simulink model "sensor_less"  (R2023a)
settings: Solver=VariableStepAuto  StartTime=0.0  StopTime=1  RelTol=1e-3
libraries: spsMosfetLib x6, slpidlib x1, spsPermanentMagnetSynchronousMachineLib x1, spsDCVoltageSourceLib x1, dspswit3 x1, spspowerguiLib x1
settings Model: Creator=heman  LastModifiedBy=ANKIT
settings SolverCC: ZeroCrossAlgorithm=Adaptive
settings DebuggingCC: IgnoredZcDiagnostic=none

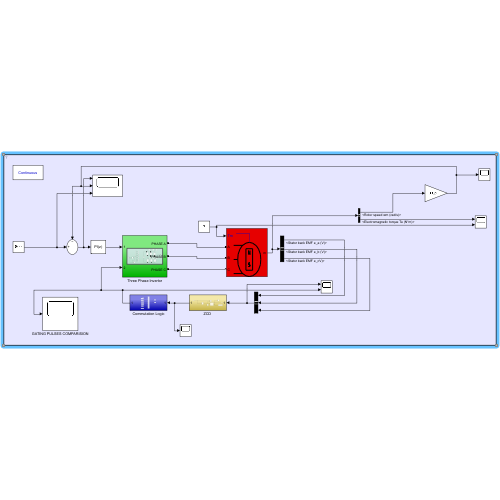
[thumbnail: Simulink's stored preview of the top-level diagram]
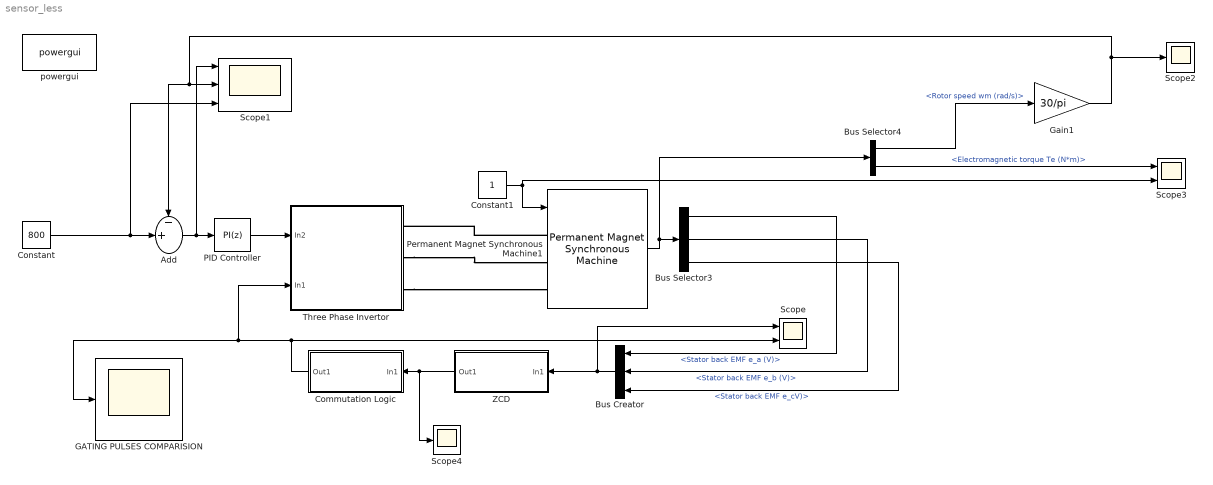
== system sensor_less ==
  Add : Sum  Inputs=-+|
  Bus Creator : BusCreator  Inputs=3
  Bus Selector3 : BusSelector  OutputSignals=Stator back EMF e_a (V),Stator back EMF e_b (V),Stator back EMF e_cV)
  Bus Selector4 : BusSelector  OutputSignals=Rotor speed wm (rad/s),Electromagnetic torque Te (N*m)
  Commutation Logic : Subsystem
  Constant : Constant  Value=800
  Constant1 : Constant
  GATING PULSES COMPARISION : Scope
  Gain1 : Gain  Gain=30/pi
  PID Controller : slpidlib/PID Controller  Controller=PI  Form=Parallel  TimeDomain=Discrete-time  UseExternalTs=off  SampleTime=-1  IntegratorMethod=Forward Euler  FilterMethod=Forward Euler  ControllerParametersSource=internal  P=0.01035  I=12.77  UseKiTs=on  D=500  N=100  UseFilter=on  TunerSelectOption=Frequency Response Based  InitialConditionSource=internal  InitialConditionForIntegrator=0  InitialConditionForFilter=0  DifferentiatorICPrevScaledInput=0  ExternalReset=none  TrackingMode=off  Kt=1  LimitOutput=off  SatLimitsSource=internal  UpperSaturationLimit=inf  LowerSaturationLimit=-inf  LinearizeAsGain=on  AntiWindupMode=none  Kb=1  LimitIntegrator=off  UpperIntegratorSaturationLimit=inf  LowerIntegratorSaturationLimit=-inf  POutMin=[]  POutMax=[]  IOutMin=[]  IOutMax=[]  DOutMin=[]  DOutMax=[]  NOutMin=[]  NOutMax=[]  SumOutMin=[]  SumOutMax=[]  SaturationOutMin=[]  SaturationOutMax=[]  PParamMin=[]  PParamMax=[]  IParamMin=[]  IParamMax=[]  DParamMin=[]  DParamMax=[]  NParamMin=[]  NParamMax=[]  KbParamMin=[]  KbParamMax=[]  KtParamMin=[]  KtParamMax=[]  KbOutMin=[]  KbOutMax=[]  KtOutMin=[]  KtOutMax=[]  IntegratorOutMin=[]  IntegratorOutMax=[]  FilterOutMin=[]  FilterOutMax=[]  SumI1OutMin=[]  SumI1OutMax=[]  SumI2OutMin=[]  SumI2OutMax=[]  SumI3OutMin=[]  SumI3OutMax=[]  SumI4OutMin=[]  SumI4OutMax=[]  SumDOutMin=[]  SumDOutMax=[]  DifferentiatorOutMin=[]  DifferentiatorOutMax=[]  FilterDiffOutCoefMin=[]  FilterDiffOutCoefMax=[]  ReciprocalOutMin=[]  ReciprocalOutMax=[]  SumDenOutMin=[]  SumDenOutMax=[]  SumNumOutMin=[]  SumNumOutMax=[]  DivideOutMin=[]  DivideOutMax=[]  UdiffTsProdOutMin=[]  UdiffTsProdOutMax=[]  NTsProdOutMin=[]  NTsProdOutMax=[]  UintegralTsProdOutMin=[]  UintegralTsProdOutMax=[]  UngainTsProdOutMin=[]  UngainTsProdOutMax=[]  ClampingZeroOutDataTypeStr=Inherit: Inherit via back propagation  ClampingZeroOutMin=[]  ClampingZeroOutMax=[]  FilterDenConstantOutDataTypeStr=Inherit: Inherit via back propagation  FilterDenConstantOutMin=[]  FilterDenConstantOutMax=[]  PCopyOutDataTypeStr=Inherit: Inherit via back propagation  PCopyOutMin=[]  PCopyOutMax=[]  NCopyOutDataTypeStr=Inherit: Inherit via back propagation  NCopyOutMin=[]  NCopyOutMax=[]  IntegratorContinuousStateAttributes=''  IntegratorStateMustResolveToSignalObject=off  IntegratorRTWStateStorageClass=Auto  FilterContinuousStateAttributes=''  FilterStateMustResolveToSignalObject=off  FilterRTWStateStorageClass=Auto  ParallelPVariant=InternalParameters  IdealPVariant=Disabled  IVariant=InternalParameters  DVariant=Disabled  IntegratorVariant=Discrete  SatVariant=Disabled  AWVariant=Passthrough  PCopyVariant=Disabled  TRVariant=Disabled  FdbkBlocksVariant=Forward  IdealPFdbkVariant=Disabled  SatFdbkVariant=Disabled  DerivativeFilterVariant=Disabled  NVariant=Disabled  NCopyVariant=Disabled_SignalSpec  FilterICVariant=Disabled  IntegratorICVariant=InternalICs  ExternalResetVariant=Disabled  TRSumVariant=Passthrough  SumFdbkVariant=Disabled  SumVariant=Sum_PI  TsampFilterVariant=InternalTs  TsampNgainVariant=Passthrough  TsampIntegralVariant=Passthrough  ExternalSaturationOutDataTypeStr=Inherit: Same as second input
  Permanent Magnet Synchronous Machine1 : spsPermanentMagnetSynchronousMachineLib/Permanent Magnet Synchronous Machine  NbPhases=3  FluxDistribution=Trapezoidal  RotorType=Round  MechanicalLoad=Torque Tm  PresetModel=No  ShowDetailedParameters=on  MeasurementBus=off  Resistance=0.7  Inductance=2.7e-3  dqInductances=[8.5e-3,8.5e-3]  La=0.000395  MachineConstant=Voltage Constant (V_peak L-L / krpm)  Flux=0.12322  VoltageCst=103.2327  TorqueCst=0.9858  Flat=120  Mechanical=[0.0027 0.0004924 4 0]  PolePairs=4  InitialConditions=[0,0, 0,0]  InitialConditions5ph=[0 0 0 0 0 0]  RefAngle=90 degrees behind phase A axis (modified Park)  IterativeDiscreteModel=Trapezoidal non iterative  TsBlock=-1  TsPowergui=0
  Scope : Scope  NumInputPorts=2
  Scope1 : Scope  NumInputPorts=3
  Scope2 : Scope
  Scope3 : Scope  NumInputPorts=2
  Scope4 : Scope
  Three Phase Invertor : Subsystem
  "ZCD " : Subsystem
  powergui : spspowerguiLib/powergui  Priority=1  SimulationMode=Continuous  SampleTime=50e-6  frequency=60  Iterations=50  frequencyindice=0  Pbase=100e6  ErrMax=1e-4  UnitsV=kV  UnitsW=MW  buscounter=0  FunctionMessages=off  echomessages=off  EnableUseOfTLC=off  CurrentSourceSwitches=off  DisableSnubberDevices=off  DisableRonSwitches=off  DisableVfSwitches=off  DisplayEquations=off  AutomaticDiscreteSolvers=off  SolverType=Tustin/Backward Euler (TBE)  Interpol=off  ExternalGateDelay=off  methode=off  Ts=100  x0status=blocks  SPID=on  SwTol=0  HookPort=off  NonlinearTolerance=0  nMaxIteration=15  ContinueOnMaxIteration=off  RestoreLinks=warning  ResistiveCurrentMeasurement=off  Frange=[0:2:500]  Ylog=off  Xlog=on  ShowGrid=off  save=off  variable=ZData  structure=0  ZoomFFT=off  StartTime=0.0  cycles=1  DisplayStyle=1  fundamental=60  FreqAxis=off  MaxFrequency=1000  frequencyindicesteady=1  RmsSteady=1  display=off
  wires:
  Constant/1 -> Scope1/3, Add/2
  Permanent Magnet Synchronous Machine1/1 -> Bus Selector4/1, Bus Selector3/1
  Bus Creator/1 -> Scope/1, "ZCD "/1(In1)
  Bus Selector3/1 -> Bus Creator/1  "<Stator back EMF e_a (V)>"
  Bus Selector3/2 -> Bus Creator/2  "<Stator back EMF e_b (V)>"
  Bus Selector3/3 -> Bus Creator/3  "<Stator back EMF e_cV)>"
  Constant1/1 -> Permanent Magnet Synchronous Machine1/1, Scope3/2
  "ZCD "/1(Out1) -> Commutation Logic/1(In1), Scope4/1
  Bus Selector4/1 -> Gain1/1  "<Rotor speed wm (rad/s)>"
  Gain1/1 -> Scope2/1, Add/1, Scope1/2
  Bus Selector4/2 -> Scope3/1  "<Electromagnetic torque Te (N*m)>"
  PID Controller/1 -> Three Phase Invertor/1(In2)
  Add/1 -> PID Controller/1, Scope1/1
  Commutation Logic/1(Out1) -> GATING PULSES COMPARISION/1, Three Phase Invertor/2(In1), Scope/2
  connections:
  Permanent Magnet Synchronous Machine1/LConn1 -- Three Phase Invertor/RConn1
  Three Phase Invertor/RConn3 -- Permanent Magnet Synchronous Machine1/LConn3
  Three Phase Invertor/RConn2 -- Permanent Magnet Synchronous Machine1/LConn2

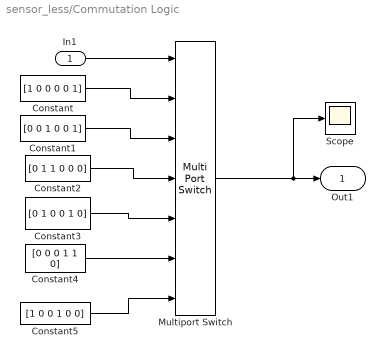
== system sensor_less/Commutation Logic ==
  In1 : Inport
  Constant : Constant  Value=[1 0 0 0 0 1]  VectorParams1D=off
  Constant1 : Constant  Value=[0 0 1 0 0 1]  VectorParams1D=off
  Constant2 : Constant  Value=[0 1 1 0 0 0]  VectorParams1D=off
  Constant3 : Constant  Value=[0 1 0 0 1 0]  VectorParams1D=off
  Constant4 : Constant  Value=[0 0 0 1 1 0]  VectorParams1D=off
  Constant5 : Constant  Value=[1 0 0 1 0 0]  VectorParams1D=off
  Multiport Switch : MultiPortSwitch  DataPortOrder=Zero-based contiguous  Inputs=6  zeroidx=on  SaturateOnIntegerOverflow=off  InputSameDT=off
  Scope : Scope
  Out1 : Outport
  wires:
  In1/1 -> Multiport Switch/1
  Multiport Switch/1 -> Scope/1, Out1/1
  Constant5/1 -> Multiport Switch/7
  Constant4/1 -> Multiport Switch/6
  Constant/1 -> Multiport Switch/2
  Constant1/1 -> Multiport Switch/3
  Constant2/1 -> Multiport Switch/4
  Constant3/1 -> Multiport Switch/5

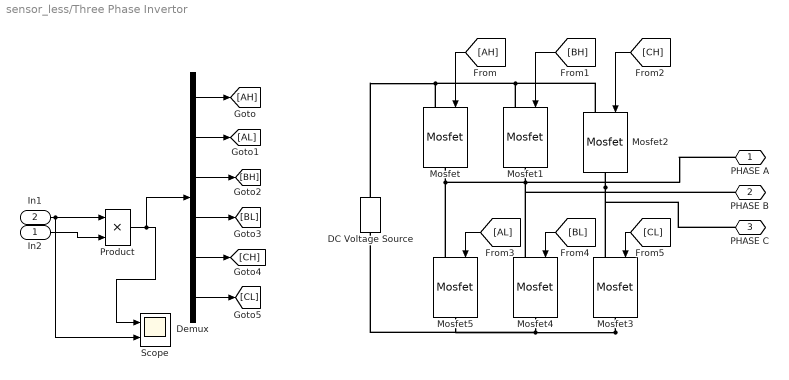
== system sensor_less/Three Phase Invertor ==
  In2 : Inport
  In1 : Inport  Port=2
  DC Voltage Source : spsDCVoltageSourceLib/DC Voltage Source  Amplitude=150  Measurements=None
  Demux : Demux  Outputs=6
  Mosfet{,1..5} (6 alike) : spsMosfetLib/Mosfet  Ron=1e-3  Lon=0  Rd=0.01  Vfd=0  IC=0  Rs=1e5  Cs=inf  Measurements=off
  Product : Product
  Scope : Scope  NumInputPorts=2
  PHASE A : PMIOPort  Side=Right
  PHASE B : PMIOPort  Port=2  Side=Right
  PHASE C : PMIOPort  Port=3  Side=Right
  wires:
  [AH] -> Mosfet/1
  [CH] -> Mosfet2/1
  [BH] -> Mosfet1/1
  [AL] -> Mosfet5/1
  [BL] -> Mosfet4/1
  [CL] -> Mosfet3/1
  Demux/1 -> [AH]
  Demux/2 -> [AL]
  Demux/3 -> [BH]
  Demux/4 -> [BL]
  Demux/5 -> [CH]
  Demux/6 -> [CL]
  In1/1 -> Scope/2, Product/1
  In2/1 -> Product/2
  Product/1 -> Demux/1, Scope/1
  connections:
  Mosfet3/RConn1 -- DC Voltage Source/LConn1 -- Mosfet5/RConn1 -- Mosfet4/RConn1
  Mosfet2/RConn1 -- Mosfet3/LConn1 -- PHASE C/RConn1
  Mosfet1/RConn1 -- PHASE B/RConn1 -- Mosfet4/LConn1
  Mosfet1/LConn1 -- Mosfet2/LConn1 -- DC Voltage Source/RConn1 -- Mosfet/LConn1
  Mosfet/RConn1 -- Mosfet5/LConn1 -- PHASE A/RConn1

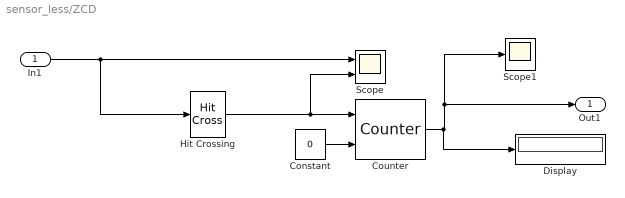
== system sensor_less/ZCD  ==
  In1 : Inport
  Constant : Constant  Value=0
  Counter : dspswit3/Counter  Direction=Up  CountEvent=Rising edge  CounterSize=User defined  MaxCount=5  InitialCount=0  Output=Count  HitValue=32  ResetInput=on  SamplesPerFrame=1  Ts=1  CntDtype=double  HitDtype=Logical
  Display : Display
  Hit Crossing : HitCross
  Scope : Scope  NumInputPorts=2
  Scope1 : Scope
  Out1 : Outport
  wires:
  In1/1 -> Scope/1, Hit Crossing/1
  Hit Crossing/1 -> Scope/2, Counter/1
  Constant/1 -> Counter/2
  Counter/1 -> Scope1/1, Out1/1, Display/1
